simulink model "Fig21"  (R2014a)
settings: Solver=ode3  StartTime=0.0  StopTime=5e-2  FixedStep=2e-5  RelTol=1e-5
libraries: commchan3 x1, commrandsrc2 x1, dspsigops x1
settings Model: Creator=Dennis Silage  LastModifiedBy=Silage
settings DataIOCC: SignalLoggingSaveFormat=ModelDataLogs
settings OptimizationCC: ExpressionDepthLimit=2147483647  InitFltsAndDblsToZero=on
settings DebuggingCC: UnderspecifiedInitializationDetection=Classic  SolverPrmCheckMsg=none  FcnCallInpInsideContextMsg=UseLocalSettings  StateNameClashWarn=warning
settings GRTTargetCC: CombineOutputUpdateFcns=off  GRTInterface=on

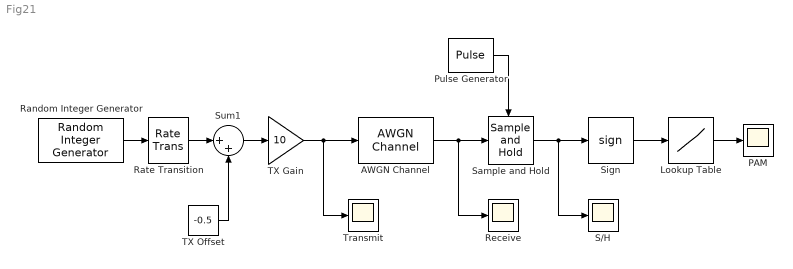
== system Fig21 ==
  AWGN Channel : commchan3/AWGN Channel  InputProcessing=Inherited (this choice will be removed - see release notes)  seed=randseed  noiseMode=Variance from mask  EbNodB=10  EsNodB=10  SNRdB=10  bitsPerSym=1  Ps=1  Tsym=1  variance=0.5
  Lookup Table : Lookup_n-D  NumberOfTableDimensions=1  BreakpointsForDimension1=[-1, 0, 1]  Table=[-5, 5, 5]  InternalRulePriority=Speed  RndMeth=Nearest  InputSameDT=on
  PAM : Scope
      settings: YMin=-8  YMax=8  SaveName=ScopeData2
  Pulse Generator : DiscretePulseGenerator  Period=50  PhaseDelay=25  SampleTime=2e-5
  Random Integer Generator : commrandsrc2/Random Integer Generator  mul=2  seed=randseed  Ts=1e-3  frameBased=off  sampPerFrame=50  orient=on  outDataType=double
  Rate Transition : RateTransition  OutPortSampleTime=2e-5
  Receive : Scope
      settings: TimeRange=0.05  YMin=-8  YMax=8  SaveName=ScopeData3
  S/H : Scope
      settings: YMin=-8  YMax=8
  Sample and Hold : dspsigops/Sample and Hold  trig=Rising edge  initCond=0  latchinput=off
  Sign : Signum
  Sum1 : Sum  Inputs=|++
  TX Gain : Gain  Gain=10
  TX Offset : Constant  Value=-0.5
  Transmit : Scope
      settings: TimeRange=0.05  YMin=-8  YMax=8
  wires:
  Pulse Generator/1 -> Sample and Hold/Trigger
  AWGN Channel/1 -> Sample and Hold/1, Receive/1
  TX Gain/1 -> AWGN Channel/1, Transmit/1
  Sign/1 -> Lookup Table/1
  Random Integer Generator/1 -> Rate Transition/1
  Rate Transition/1 -> Sum1/1
  Sum1/1 -> TX Gain/1
  TX Offset/1 -> Sum1/2
  Sample and Hold/1 -> Sign/1, S/H/1
  Lookup Table/1 -> PAM/1
